simulink model "APSv3"  (R2020b)
settings: Solver=FixedStepDiscrete  StartTime=0.0  StopTime=Tmax  FixedStep=Ts  RelTol=1e-3
PreLoadFcn:
  | ROSconfig
  | wptsSignalSetup
PostLoadFcn:
  | configParameters
InitFcn:
  | configParameters
StartFcn:
  | gazeboSetup
StopFcn:
  | gazeboReset
  | goalreset
  | loadResults
model workspace (MAT data in the model file):
  idx = 1
  y : Simulink.Parameter (value not decoded)
values from neighbouring files (symbols this model uses):
  distError = sqrt((initX^2)+(initY^2))    [config_APS_Turb.m]
  dynamicPlume = 0    [config_APS_Turb.m]
  init = [initX - 5,initY]    [config_APS_Turb.m]
  MaxC = max(max(max(PlumeD)))    [config_APS_Turb.m]
  N = 8    [config_APS_Turb.m]
  n = [n; i*(2*pi/N)]    [config_APS_Turb.m]
  Res = 1    [config_APS_Turb.m]
  Shrink = 1/Expand    [config_APS_Turb.m]
undefined symbols (not defined in the file or in its folder): angmax, Angular, concDetectionAccuracy, DiscIntNeverNeededParam, distThresh, Expand, get, hot, Kd, Ki, Kp, LimitSize, Linear, OffsetY, PlumeD, ResX, ResY, sensorDist, sourceAccuracy, T, Tmax, Ts, vmax, wgain
libraries: simulink x18, dspindex x8, dspswit3 x6, robotlib x3, dspsnks4 x3, sm_lib x2, nesl_utility x1, dspsigops x1, mobileRoboticsLib x1
(part 2 of 2)

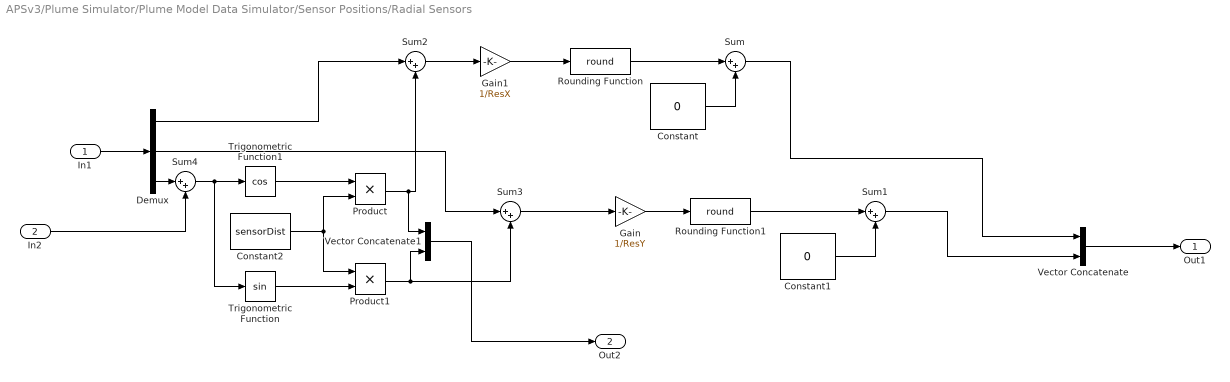
== system APSv3/Plume Simulator/Plume Model Data Simulator/Sensor Positions/Radial Sensors ==
  In1 : Inport
  In2 : Inport  Port=2
  Constant : Constant  Value=0
  Constant1 : Constant  Value=0
  Constant2 : Constant  Value=sensorDist
  Demux : Demux  Outputs=3
  Gain : Gain  Gain=1/ResY
  Gain1 : Gain  Gain=1/ResX
  Product : Product
  Product1 : Product
  Rounding Function : Rounding  Operator=round
  Rounding Function1 : Rounding  Operator=round
  Sum{,1..4} (5 alike) : Sum  Inputs=|++
  Trigonometric Function : Trigonometry
  Trigonometric Function1 : Trigonometry  Operator=cos
  Vector Concatenate : Concatenate
  Vector Concatenate1 : Concatenate
  Out1 : Outport  VectorParamsAs1DForOutWhenUnconnected=off
  Out2 : Outport  Port=2  VectorParamsAs1DForOutWhenUnconnected=off
  wires:
  Product/1 -> Vector Concatenate1/1, Sum2/2
  Sum2/1 -> Gain1/1
  Vector Concatenate/1 -> Out1/1
  Sum4/1 -> Trigonometric Function/1, Trigonometric Function1/1
  Demux/1 -> Sum2/1
  Vector Concatenate1/1 -> Out2/1
  Trigonometric Function/1 -> Product1/2
  In1/1 -> Demux/1
  Product1/1 -> Vector Concatenate1/2, Sum3/2
  In2/1 -> Sum4/2
  Constant1/1 -> Sum1/2
  Rounding Function1/1 -> Sum1/1
  Sum3/1 -> Gain/1
  Gain1/1 -> Rounding Function/1
  Gain/1 -> Rounding Function1/1
  Rounding Function/1 -> Sum/1
  Constant/1 -> Sum/2
  Sum/1 -> Vector Concatenate/1
  Sum1/1 -> Vector Concatenate/2
  Trigonometric Function1/1 -> Product/1
  Demux/3 -> Sum4/1
  Demux/2 -> Sum3/1
  Constant2/1 -> Product1/1, Product/2

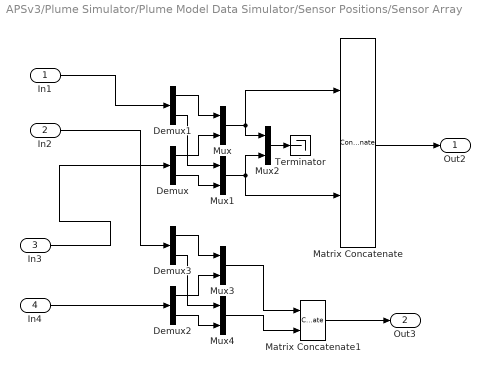
== system APSv3/Plume Simulator/Plume Model Data Simulator/Sensor Positions/Sensor Array ==
  In1 : Inport
  In2 : Inport  Port=2
  In3 : Inport  Port=3
  In4 : Inport  Port=4
  Demux{,1..3} (4 alike) : Demux  Outputs=2
  Matrix Concatenate : Concatenate  Mode=Multidimensional array  ConcatenateDimension=2
  Matrix Concatenate1 : Concatenate  Mode=Multidimensional array  ConcatenateDimension=2
  Mux{,1..4} (5 alike) : Mux  Inputs=2
  Terminator : Terminator
  Out2 : Outport  VectorParamsAs1DForOutWhenUnconnected=off
  Out3 : Outport  Port=2  VectorParamsAs1DForOutWhenUnconnected=off
  wires:
  Mux2/1 -> Terminator/1
  In1/1 -> Demux1/1
  Demux1/1 -> Mux/1
  Demux/1 -> Mux/2
  Demux1/2 -> Mux1/1
  Demux/2 -> Mux1/2
  Mux/1 -> Matrix Concatenate/1, Mux2/1
  Mux1/1 -> Mux2/2, Matrix Concatenate/2
  Matrix Concatenate/1 -> Out2/1
  Matrix Concatenate1/1 -> Out3/1
  In2/1 -> Demux3/1
  Demux3/1 -> Mux3/1
  Demux2/1 -> Mux3/2
  Demux3/2 -> Mux4/1
  Demux2/2 -> Mux4/2
  In4/1 -> Demux2/1
  Mux3/1 -> Matrix Concatenate1/1
  Mux4/1 -> Matrix Concatenate1/2
  In3/1 -> Demux/1

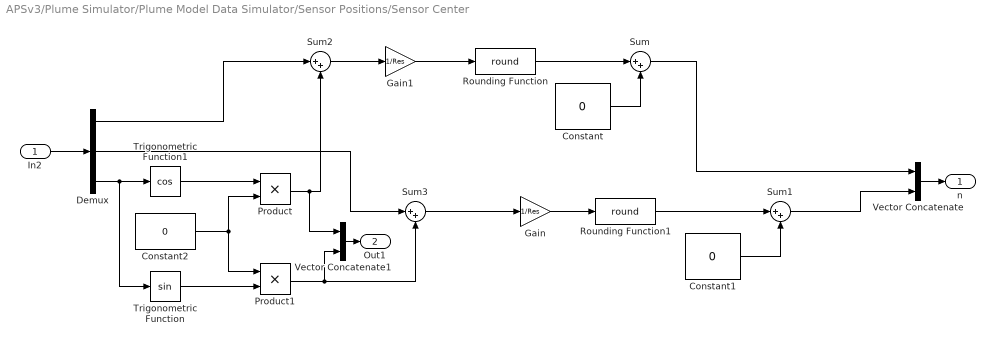
== system APSv3/Plume Simulator/Plume Model Data Simulator/Sensor Positions/Sensor Center ==
  In2 : Inport
  Constant : Constant  Value=0
  Constant1 : Constant  Value=0
  Constant2 : Constant  Value=0
  Demux : Demux  Outputs=3
  Gain : Gain  Gain=1/Res
  Gain1 : Gain  Gain=1/Res
  Product : Product
  Product1 : Product
  Rounding Function : Rounding  Operator=round
  Rounding Function1 : Rounding  Operator=round
  Sum{,1..3} (4 alike) : Sum  Inputs=|++
  Trigonometric Function : Trigonometry
  Trigonometric Function1 : Trigonometry  Operator=cos
  Vector Concatenate : Concatenate
  Vector Concatenate1 : Concatenate
  n : Outport  VectorParamsAs1DForOutWhenUnconnected=off
  Out1 : Outport  Port=2  VectorParamsAs1DForOutWhenUnconnected=off
  wires:
  Rounding Function/1 -> Sum/1
  Rounding Function1/1 -> Sum1/1
  Constant/1 -> Sum/2
  Constant1/1 -> Sum1/2
  Sum/1 -> Vector Concatenate/1
  Sum1/1 -> Vector Concatenate/2
  Gain1/1 -> Rounding Function/1
  Gain/1 -> Rounding Function1/1
  Sum2/1 -> Gain1/1
  Sum3/1 -> Gain/1
  In2/1 -> Demux/1
  Demux/1 -> Sum2/1
  Demux/2 -> Sum3/1
  Demux/3 -> Trigonometric Function/1, Trigonometric Function1/1
  Constant2/1 -> Product1/1, Product/2
  Product/1 -> Vector Concatenate1/1, Sum2/2
  Product1/1 -> Vector Concatenate1/2, Sum3/2
  Vector Concatenate/1 -> n/1
  Trigonometric Function1/1 -> Product/1
  Trigonometric Function/1 -> Product1/2
  Vector Concatenate1/1 -> Out1/1

== matlab function APSv3/Odometry Subscriber/Odometry Conversion/Conversion ==
  data: yaw output; x input; y input; z input; w input
function yaw  = quat2eul(x,y,z,w)
%#codegen

% Convert the quaternion to a yaw angle (zyx euler angle)
eul = quat2eul([w,x,y,z]);
yaw = eul(1);

end

== matlab function APSv3/Plume Simulator/Plume Model Data Simulator/Static Plume Concentrations/MATLAB Function ==
  data: PlumeD input; Plume output; Peak output; OffsetY input
function [Plume, Peak] = fcn(PlumeD,OffsetY)

%Plume = squeeze(PlumeD(:,:,u));

%Plume = PlumeD(:,:,u);
Plume = PlumeD(:,:);

Cmax = max(max(Plume(:)));

Peak = [1 OffsetY+1];

end

function coord = maxmat( c )
as=size(c);
total_ele=numel(c);
[~,I]=max(c(:));
r=rem(I,as(1));
a=r;
b=((I-a)/as(1))+1;
if a==0
    a=as(1);
    b=b-1;
else
    a=r;
    b=b;
end

coord = [b,a]

end

== matlab function APSv3/Removed Blocks/Dynamic Plume Concentrations/MATLAB Function ==
  data: PlumeD input; u input; Plume output; Cmax output; Peak output; OffsetY input
function [Plume, Cmax, Peak] = fcn(PlumeD,u,OffsetY)

%Plume = squeeze(PlumeD(:,:,u));

%Plume = PlumeD(:,:,u);
Plume = PlumeD(:,:);

Cmax = max(max(Plume(:)));

Peak = [1 OffsetY+1];

end

function coord = maxmat( c )
as=size(c);
total_ele=numel(c);
[~,I]=max(c(:));
r=rem(I,as(1));
a=r;
b=((I-a)/as(1))+1;
if a==0
    a=as(1);
    b=b-1;
else
    a=r;
    b=b;
end

coord = [b,a]

end

== matlab function APSv3/Plume Simulator/Plume Model Data Simulator/Sensor Data Matrix/MATLAB Function ==
  data: plume input; cMap input; poses input; N input; Cdata data_store_memory size=[(N+1) 1]; Cdata1 output size=N+1; offY input; cMap1 output; maxPose data_store_memory size=2; MaxPose output size=2
function [Cdata1,cMap1,MaxPose]= fcn(plume,cMap,poses,N,offY)

Cdata = zeros(N,1);
Cdata1 = zeros(N,1);
cMap1 = zeros(size(plume,1),size(plume,2));

%coder.varsize('maxPose');
%Phi = PhiInput;
MaxPose = zeros(2,1);
maxPose = zeros(2,1);

for i = 1:N
    if poses(i,1) < 1
    poses(i,1) = 1;
    elseif poses(i,2) == 0
    poses(i,2) = 1;
    end

    cols = plume(:,poses(i,1));
    rows = cols(poses(i,2)+offY,1);
    
    Cdata(i) = rows(1);
    cMap(poses(i,2)+offY,poses(i,1)) = rows(1);
    
end

    cMap1 = cMap(:,:);
    Cdata1 = Cdata;
    
    p = find(Cdata1 == max(Cdata1));
    
    if size(p,1) == 1 
        %if size(poses,1) > 1
            maxPose(:,:) = [poses(p,1); poses(p,2)];
            %maxPose(1) = poses(p,1);
            %maxPose(2) = poses(p,2);
        %end
    else
        maxPose = [poses(1,1); poses(1,2)];
        %maxPose = [1; 1];
    end
    
    MaxPose = maxPose;

end
